simulink model "threeservos"  (Simulink 8.3)
settings: Solver=ode45  StartTime=0.0  StopTime=1  RelTol=1e-3
InitFcn:
  | clear functions
settings Model: Creator=anton  LastModifiedBy=matteo  ExtModeTrigMode=oneshot  ExtModeArmWhenConnect=off  ExtModeAutoUpdateStatusClock=off
settings DataIOCC: LimitDataPoints=off
settings OptimizationCC: BlockReduction=off  BooleanDataType=off  InlineParams=on  ExpressionDepthLimit=2147483647
settings DebuggingCC: SaveWithParameterizedLinksMsg=none  SignalResolutionControl=TryResolveAllWithWarning  SolverPrmCheckMsg=none  MultiTaskDSMMsg=warning  MultiTaskCondExecSysMsg=none  FcnCallInpInsideContextMsg=UseLocalSettings  StrictBusMsg=None
settings HardwareCC: TargetUnknown=on
settings RTWCC: IncludeERTFirstTime=on

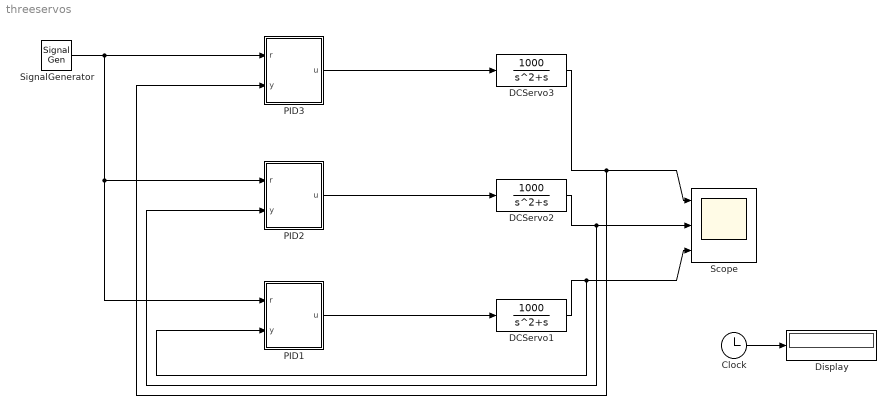
== system threeservos ==
  Clock : Clock
  DCServo1 : TransferFcn  Numerator=[1000]  Denominator=[1 1 0]
  DCServo2 : TransferFcn  Numerator=[1000]  Denominator=[1 1 0]
  DCServo3 : TransferFcn  Numerator=[1000]  Denominator=[1 1 0]
  Display : Display
  PID1 : Subsystem  mask{K=0.96, Ti=0.12, Td=0.049, beta=0.5, N=10, h=0.006}
  PID2 : Subsystem  mask{K=0.96, Ti=0.12, Td=0.049, beta=0.5, N=10, h=0.005}
  PID3 : Subsystem  mask{K=0.96, Ti=0.12, Td=0.049, beta=0.5, N=10, h=0.004}
  Scope : Scope  NumInputPorts=3
      settings: YMin=-5~-5~-5  YMax=5~5~5
  SignalGenerator : SignalGenerator  WaveForm=square  Frequency=1.5
  wires:
  Clock/1 -> Display/1
  SignalGenerator/1 -> PID1/1(r), PID2/1(r), PID3/1(r)
  DCServo3/1 -> Scope/1, PID3/2(y)
  DCServo2/1 -> Scope/2, PID2/2(y)
  DCServo1/1 -> Scope/3, PID1/2(y)
  PID3/1(u) -> DCServo3/1
  PID2/1(u) -> DCServo2/1
  PID1/1(u) -> DCServo1/1

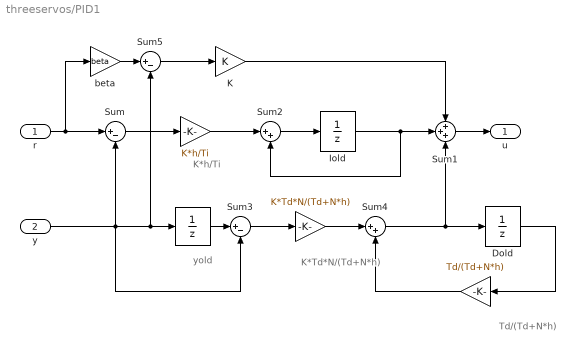
== system threeservos/PID1 ==
  note: K*h/Ti
  note: K*Td*N/(Td+N*h)
  note: Td/(Td+N*h)
  note: yold
  r : Inport
  y : Inport  Port=2
  " " : UnitDelay  SampleTime=h
  "   " : Gain  Gain=K*h/Ti  SaturateOnIntegerOverflow=on  OutDataTypeStr=Inherit: Same as input  ParamDataTypeStr=Inherit: Same as input
  "             " : Gain  Gain=K*Td*N/(Td+N*h)  SaturateOnIntegerOverflow=on  OutDataTypeStr=Inherit: Same as input  ParamDataTypeStr=Inherit: Same as input
  "              " : Gain  Gain=Td/(Td+N*h)  SaturateOnIntegerOverflow=on  OutDataTypeStr=Inherit: Same as input  ParamDataTypeStr=Inherit: Same as input
  Dold : UnitDelay  SampleTime=h
  "Iold " : UnitDelay  SampleTime=h
  K : Gain  Gain=K  SaturateOnIntegerOverflow=on  OutDataTypeStr=Inherit: Same as input  ParamDataTypeStr=Inherit: Same as input
  Sum : Sum  Inputs=|+-  SaturateOnIntegerOverflow=on  InputSameDT=on  OutDataTypeStr=Inherit: Same as first input
  Sum1 : Sum  Inputs=+++  SaturateOnIntegerOverflow=on  InputSameDT=on  OutDataTypeStr=Inherit: Same as first input
  Sum2 : Sum  Inputs=|++  SaturateOnIntegerOverflow=on  InputSameDT=on  OutDataTypeStr=Inherit: Same as first input
  Sum3 : Sum  Inputs=|+-  SaturateOnIntegerOverflow=on  InputSameDT=on  OutDataTypeStr=Inherit: Same as first input
  Sum4 : Sum  Inputs=|++  SaturateOnIntegerOverflow=on  InputSameDT=on  OutDataTypeStr=Inherit: Same as first input
  Sum5 : Sum  Inputs=|+-  SaturateOnIntegerOverflow=on  InputSameDT=on  OutDataTypeStr=Inherit: Same as first input
  beta : Gain  Gain=beta  SaturateOnIntegerOverflow=on  OutDataTypeStr=Inherit: Same as input  ParamDataTypeStr=Inherit: Same as input
  u : Outport
  wires:
  y/1 -> Sum/2, Sum3/2, " "/1, Sum5/2
  r/1 -> Sum/1, beta/1
  Sum1/1 -> u/1
  K/1 -> Sum1/1
  Sum2/1 -> "Iold "/1
  Dold/1 -> "              "/1
  "             "/1 -> Sum4/1
  Sum3/1 -> "             "/1
  Sum4/1 -> Dold/1, Sum1/3
  " "/1 -> Sum3/1
  "Iold "/1 -> Sum2/2, Sum1/2
  "   "/1 -> Sum2/1
  Sum/1 -> "   "/1
  "              "/1 -> Sum4/2
  beta/1 -> Sum5/1
  Sum5/1 -> K/1

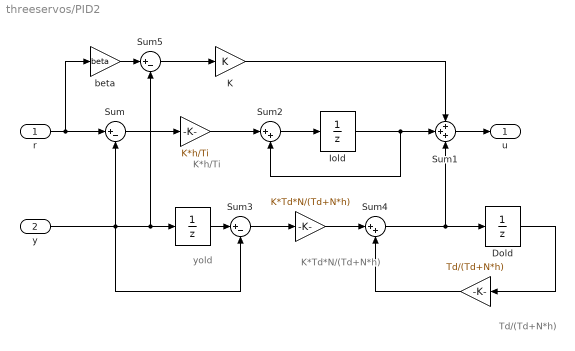
== system threeservos/PID2 ==
  note: K*h/Ti
  note: K*Td*N/(Td+N*h)
  note: Td/(Td+N*h)
  note: yold
  r : Inport
  y : Inport  Port=2
  " " : UnitDelay  SampleTime=h
  "   " : Gain  Gain=K*h/Ti  SaturateOnIntegerOverflow=on  OutDataTypeStr=Inherit: Same as input  ParamDataTypeStr=Inherit: Same as input
  "             " : Gain  Gain=K*Td*N/(Td+N*h)  SaturateOnIntegerOverflow=on  OutDataTypeStr=Inherit: Same as input  ParamDataTypeStr=Inherit: Same as input
  "              " : Gain  Gain=Td/(Td+N*h)  SaturateOnIntegerOverflow=on  OutDataTypeStr=Inherit: Same as input  ParamDataTypeStr=Inherit: Same as input
  Dold : UnitDelay  SampleTime=h
  "Iold " : UnitDelay  SampleTime=h
  K : Gain  Gain=K  SaturateOnIntegerOverflow=on  OutDataTypeStr=Inherit: Same as input  ParamDataTypeStr=Inherit: Same as input
  Sum : Sum  Inputs=|+-  SaturateOnIntegerOverflow=on  InputSameDT=on  OutDataTypeStr=Inherit: Same as first input
  Sum1 : Sum  Inputs=+++  SaturateOnIntegerOverflow=on  InputSameDT=on  OutDataTypeStr=Inherit: Same as first input
  Sum2 : Sum  Inputs=|++  SaturateOnIntegerOverflow=on  InputSameDT=on  OutDataTypeStr=Inherit: Same as first input
  Sum3 : Sum  Inputs=|+-  SaturateOnIntegerOverflow=on  InputSameDT=on  OutDataTypeStr=Inherit: Same as first input
  Sum4 : Sum  Inputs=|++  SaturateOnIntegerOverflow=on  InputSameDT=on  OutDataTypeStr=Inherit: Same as first input
  Sum5 : Sum  Inputs=|+-  SaturateOnIntegerOverflow=on  InputSameDT=on  OutDataTypeStr=Inherit: Same as first input
  beta : Gain  Gain=beta  SaturateOnIntegerOverflow=on  OutDataTypeStr=Inherit: Same as input  ParamDataTypeStr=Inherit: Same as input
  u : Outport
  wires:
  y/1 -> Sum/2, Sum3/2, " "/1, Sum5/2
  r/1 -> Sum/1, beta/1
  Sum1/1 -> u/1
  K/1 -> Sum1/1
  Sum2/1 -> "Iold "/1
  Dold/1 -> "              "/1
  "             "/1 -> Sum4/1
  Sum3/1 -> "             "/1
  Sum4/1 -> Dold/1, Sum1/3
  " "/1 -> Sum3/1
  "Iold "/1 -> Sum2/2, Sum1/2
  "   "/1 -> Sum2/1
  Sum/1 -> "   "/1
  "              "/1 -> Sum4/2
  beta/1 -> Sum5/1
  Sum5/1 -> K/1

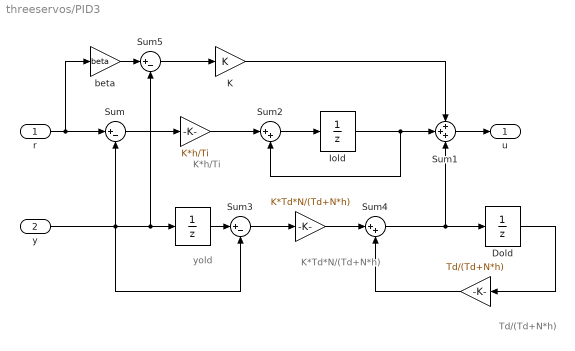
== system threeservos/PID3 ==
  note: K*h/Ti
  note: K*Td*N/(Td+N*h)
  note: Td/(Td+N*h)
  note: yold
  r : Inport
  y : Inport  Port=2
  " " : UnitDelay  SampleTime=h
  "   " : Gain  Gain=K*h/Ti  SaturateOnIntegerOverflow=on  OutDataTypeStr=Inherit: Same as input  ParamDataTypeStr=Inherit: Same as input
  "             " : Gain  Gain=K*Td*N/(Td+N*h)  SaturateOnIntegerOverflow=on  OutDataTypeStr=Inherit: Same as input  ParamDataTypeStr=Inherit: Same as input
  "              " : Gain  Gain=Td/(Td+N*h)  SaturateOnIntegerOverflow=on  OutDataTypeStr=Inherit: Same as input  ParamDataTypeStr=Inherit: Same as input
  Dold : UnitDelay  SampleTime=h
  "Iold " : UnitDelay  SampleTime=h
  K : Gain  Gain=K  SaturateOnIntegerOverflow=on  OutDataTypeStr=Inherit: Same as input  ParamDataTypeStr=Inherit: Same as input
  Sum : Sum  Inputs=|+-  SaturateOnIntegerOverflow=on  InputSameDT=on  OutDataTypeStr=Inherit: Same as first input
  Sum1 : Sum  Inputs=+++  SaturateOnIntegerOverflow=on  InputSameDT=on  OutDataTypeStr=Inherit: Same as first input
  Sum2 : Sum  Inputs=|++  SaturateOnIntegerOverflow=on  InputSameDT=on  OutDataTypeStr=Inherit: Same as first input
  Sum3 : Sum  Inputs=|+-  SaturateOnIntegerOverflow=on  InputSameDT=on  OutDataTypeStr=Inherit: Same as first input
  Sum4 : Sum  Inputs=|++  SaturateOnIntegerOverflow=on  InputSameDT=on  OutDataTypeStr=Inherit: Same as first input
  Sum5 : Sum  Inputs=|+-  SaturateOnIntegerOverflow=on  InputSameDT=on  OutDataTypeStr=Inherit: Same as first input
  beta : Gain  Gain=beta  SaturateOnIntegerOverflow=on  OutDataTypeStr=Inherit: Same as input  ParamDataTypeStr=Inherit: Same as input
  u : Outport
  wires:
  y/1 -> Sum/2, Sum3/2, " "/1, Sum5/2
  r/1 -> Sum/1, beta/1
  Sum1/1 -> u/1
  K/1 -> Sum1/1
  Sum2/1 -> "Iold "/1
  Dold/1 -> "              "/1
  "             "/1 -> Sum4/1
  Sum3/1 -> "             "/1
  Sum4/1 -> Dold/1, Sum1/3
  " "/1 -> Sum3/1
  "Iold "/1 -> Sum2/2, Sum1/2
  "   "/1 -> Sum2/1
  Sum/1 -> "   "/1
  "              "/1 -> Sum4/2
  beta/1 -> Sum5/1
  Sum5/1 -> K/1
